simulink model "exercicio"  (R2018a)
settings: Solver=VariableStepAuto  StartTime=0.0  StopTime=0.05  RelTol=1e-3
libraries: dsparch4 x1, simulink x1, dspsigops x1
settings Model: Creator=mylen  LastModifiedBy=mylen

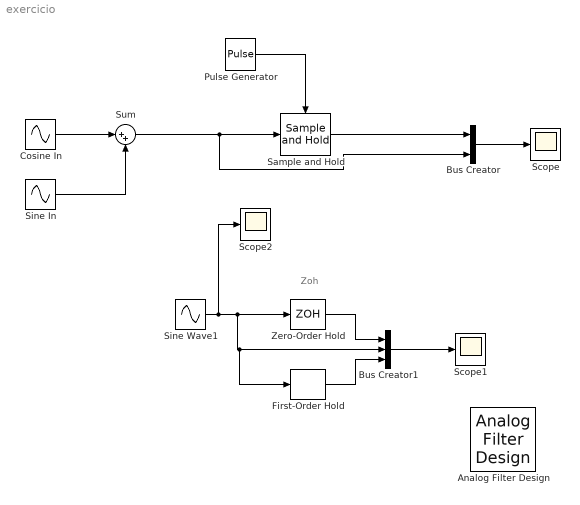
== system exercicio ==
  note: Zoh
  Analog Filter Design : dsparch4/Analog Filter Design  method=Butterworth  filttype=Lowpass  N=8  Wlo=30  Whi=80  Rp=2  Rs=40
  Bus Creator : BusCreator  Inputs=2
  Bus Creator1 : BusCreator  Inputs=3
  Cosine In : Sin  Frequency=2*pi*10  Phase=pi/2  SampleTime=0
  First-Order Hold : simulink/Discrete/First-Order Hold  DisableCoverage=on  Ts=1e-3
      settings: SourceProductName=Simulink  SourceProductBaseCode=SL
  Pulse Generator : DiscretePulseGenerator  PulseType=Time based  Period=1e-3  PulseWidth=50
  Sample and Hold : dspsigops/Sample and Hold  trig=Rising edge  initCond=0  latchinput=off
  Scope : Scope
  Scope1 : Scope
  Scope2 : Scope
  Sine In : Sin  Amplitude=0.5  Frequency=2*pi*50  Phase=pi/4  SampleTime=0
  Sine Wave1 : Sin  SineType=Sample based  SampleTime=1e-3
  Sum : Sum  Inputs=|++
  Zero-Order Hold : ZeroOrderHold  SampleTime=1e-3
  wires:
  Pulse Generator/1 -> Sample and Hold/Trigger
  Sine Wave1/1 -> Scope2/1, First-Order Hold/1, Bus Creator1/2, Zero-Order Hold/1
  Zero-Order Hold/1 -> Bus Creator1/1
  Bus Creator1/1 -> Scope1/1
  Bus Creator/1 -> Scope/1
  Sample and Hold/1 -> Bus Creator/1
  First-Order Hold/1 -> Bus Creator1/3
  Cosine In/1 -> Sum/1
  Sine In/1 -> Sum/2
  Sum/1 -> Bus Creator/2, Sample and Hold/1
